simulink model "modelo"  (R2025b)
settings: Solver=ode15s  StartTime=0.0  StopTime=15  RelTol=1e-8
undefined symbols (not defined in the file): X, Y, Z
libraries: sm_lib x30, nesl_utility x2
(part 2 of 2)

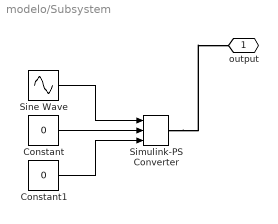
== system modelo/Subsystem ==
  Constant : Constant  Value=0
  Constant1 : Constant  Value=0
  Simulink-PS Converter : nesl_utility/Simulink-PS Converter  PhysicalDomain=network_engine_domain  SubClassName=ps_input  LeftPortType=input  RightPortType=output  PseudoPeriodic=off  Frequencies=[]  NoiseDistribution=none  NoiseParameters=[]  Unit=1  AffineConversion=off  FilteringAndDerivatives=provide  SimscapeFilterOrder=1  InputFilterTimeConstant=0.001  UdotUserProvided=2
  Sine Wave : Sin  Amplitude=0.5  SampleTime=0
  output : PMIOPort  Side=Right
  wires:
  Constant/1 -> Simulink-PS Converter/2
  Sine Wave/1 -> Simulink-PS Converter/1
  Constant1/1 -> Simulink-PS Converter/3
  connections:
  Simulink-PS Converter/RConn1 -- output/RConn1
